simulink model "RLC_Impulsion"  (R2024a)
settings: Solver=VariableStepAuto  StartTime=0.0  StopTime=0.5  MaxStep=0.0001  RelTol=1e-3
model workspace (MAT data in the model file):
  C = 0.001
  L = 10
  R = 400
settings Model: Creator=hp  LastModifiedBy=NB
settings SolverCC: AlgebraicLoopSolver=TrustRegion
settings DataIOCC: ReturnWorkspaceOutputs=off
settings DebuggingCC: UnconnectedInputMsg=warning  UnconnectedOutputMsg=warning  UnconnectedLineMsg=warning  ArithmeticOperatorsInVariantConditions=warning
settings ModelReferenceCC: EnableRefExpFcnMdlSchedulingChecks=on
settings SFSimCC: CustomCodeUndefinedFunction=UseInterfaceOnly
settings RTWCC: GPUComputeCapability=3.5

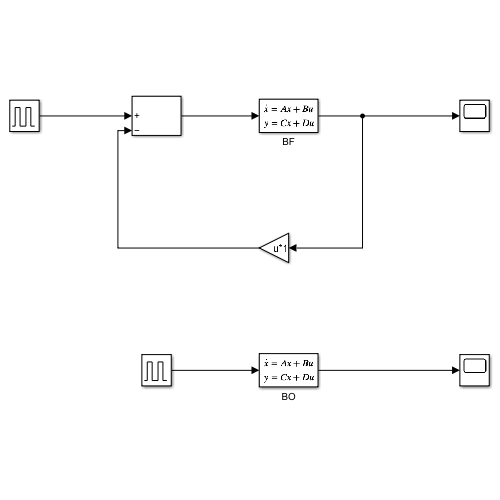
[thumbnail: Simulink's stored preview of the top-level diagram]
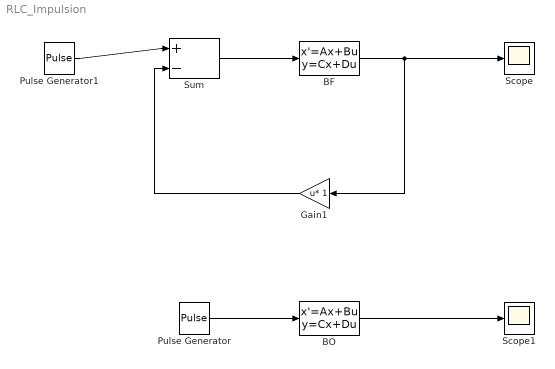
== system RLC_Impulsion ==
  BF : StateSpace  A=[-40, 0, -0.1 ; 1, 0, 0 ; 10000, 0, 0]  B=[0.1 ; 0 ; 0]  C=[0 0 1]  D=0  InitialCondition=0
  BO : StateSpace  A=[-40, 0, -0.1 ; 1, 0, 0 ; 10000, 0, 0]  B=[0.1 ; 0 ; 0]  C=[0 0 1]  D=0  InitialCondition=0
  Gain1 : Gain  Multiplication=Matrix(u*K)
  Pulse Generator : DiscretePulseGenerator  PulseType=Time based  Amplitude=1000  Period=10  PulseWidth=0.01
  Pulse Generator1 : DiscretePulseGenerator  PulseType=Time based  Amplitude=1000  Period=10  PulseWidth=0.01
  Scope : Scope
  Scope1 : Scope
  Sum : Sum  Inputs=|+-
  wires:
  Sum/1 -> BF/1
  BF/1 -> Gain1/1, Scope/1
  Gain1/1 -> Sum/2
  BO/1 -> Scope1/1
  Pulse Generator1/1 -> Sum/1
  Pulse Generator/1 -> BO/1
